simulink model "Drone2_simulink"  (R2024a)
settings: Solver=ode1be  StartTime=0.0  StopTime=1000  FixedStep=0.001  MaxStep=0.001  MinStep=0.00095  RelTol=1e-3
PreLoadFcn:
  | Drone_data;
model workspace: external: MATLAB File C:\Users\admin\OneDrive - Indian Institute of Technology Jodhpur\IIT JODHPUR\Research Work\Amphibious Drone\MATLAB_CODE\2025\New_Drone\Drone_1\Drone1_simulink_DataFile.m (data not in the file)
undefined symbols (not defined in the file): Environment, Newton, Raphson, Vehicle, X, Y, Z
libraries: sm_lib x1684, nesl_utility x63, slpidlib x25, eeGeneralControl x6, matrix_library x3, rllib x2, simulink x2, fl_lib x1, sharedutil x1, SignalEditorBlockLib x1
(part 4 of 17)

== system Drone2_simulink/Physical_system/Hydro Forces & Moments ==
  Bus Element In1 : Inport  PortName=HydroForces  Element=Drag.Forces
  Bus Element In2 : Inport  PortName=HydroForces  Element=Drag.Moments
  Bus Element In : Inport  PortName=HydroForces  Element=BuoyancyForce
  Bus Element In5 : Inport  PortName=HydroForces  Element=AddedMass.AMForcesXYZ
  Bus Element In6 : Inport  PortName=HydroForces  Element=AddedMass.AMMomentsXYZ
  Bus Element In7 : Inport  PortName=HydroForces  Element=AddedMass.CForcesXYZ
  Bus Element In8 : Inport  PortName=HydroForces  Element=AddedMass.CMomentsXYZ
  Bus Element In9 : Inport  PortName=HydroForces  Element=OceanCurrentForce
  Bus Element In11 : Inport  PortName=HydroForces  Element=WindForce
  Bus Element In10 : Inport  Port=2  PortName=CenterofMass  Element=Body.COM
  Added Mass Coriolis : Subsystem
  Added Mass Forces : Subsystem
  Buoyancy Force : Subsystem
  Lift and Drag Forces : Subsystem
  OceanCurrent Force : Subsystem
  Scope : Scope
  Scope1 : Scope
  Sum : Sum  Commented=on  Inputs=+++++
  Sum1 : Sum  Commented=on  Inputs=++++
  Wind force : Subsystem
  CoM : PMIOPort  Side=Left
  CoB : PMIOPort  Port=2  Side=Left
  wires:
  Bus Element In/1 -> Buoyancy Force/1(B)
  Bus Element In1/1 -> Sum/2, Lift and Drag Forces/1(Fxyz)
  Bus Element In2/1 -> Sum1/2, Lift and Drag Forces/3(Mxyz)
  Bus Element In5/1 -> Sum/3, Added Mass Forces/1(Fxyz)
  Bus Element In8/1 -> Sum1/4, Added Mass Coriolis/3(Mxyz)
  Bus Element In9/1 -> Sum/5, OceanCurrent Force/1(Ocean Current)
  Bus Element In10/1 -> Lift and Drag Forces/2(Centerofmass), Added Mass Coriolis/2(Centerofmass), Added Mass Forces/2(Centerofmass)
  Bus Element In6/1 -> Sum1/3, Added Mass Forces/3(Mxyz)
  Bus Element In7/1 -> Sum/4, Added Mass Coriolis/1(Fxyz)
  Bus Element In11/1 -> Wind force/1(Ocean Current)
  Sum/1 -> Scope/1
  Sum1/1 -> Scope1/1
  connections:
  CoB/RConn1 -- Buoyancy Force/RConn1
  Wind force/RConn1 -- OceanCurrent Force/RConn1 -- Added Mass Coriolis/RConn1 -- Added Mass Forces/RConn1 -- CoM/RConn1 -- Lift and Drag Forces/RConn1

== system Drone2_simulink/Physical_system/World ==
  Bottom floor : Subsystem  mask{ZB=-10, X=25, Z=0.1, Y=25, C1R=0.600, C1G=1, C1B=1.0, C2R=0, C2G=0.4, C2B=0.6}
      mask prompts: ZB "Distance of Bottom from World"; X "Length"; Z "Thikness"; Y "Width"; C1R "Red"; C1G "Green"; C1B "Blue"; C2R "Red"; C2G "Green"; C2B "Blue"
      mask init:
      | Color1 = [C1R C1G C1B];
      | Color2 = [C2R C2G C2B];
      mask DialogControl ParameterGroupVar Prompt: Bottom surface data
      mask DialogControl Container8 Prompt: Distance from World to Bottom
      mask DialogControl Container6 Prompt: Data of Each tiles
      mask DialogControl Container7 Prompt: Color 1
      mask DialogControl Container5 Prompt: Color2
      mask Display:
      | patch([0 10 10 0], [0 0 10 10], Color1);
      | patch([10 20 20 10], [0 0 10 10], Color2);
      | patch([0 10 10 0], [10 10 20 20], Color2);
      | patch([10 20 20 10], [10 10 20 20], Color1);
  MechanismConfiguration : sm_lib/Utilities/Mechanism Configuration  UniformGravity=Constant  GravityVector=[0 0 Environment.gravity]  GravityVectorUnits=m/s^2  LinearizationDelta=0.001  JointModeTransitionNonlinearIterations=2
  Solver Configuration : nesl_utility/Solver Configuration  PhysicalDomain=network_engine_domain  SubClassName=solver  LeftPortType=input  RightPortType=generic  Tones=[]  Harmonics=[]  SimulateNoise=off  Profile=off  UseLocalSampling=off  EnableSwitchedLinearOptims=on  FrequencyDomain=off  UseCCode=off  RelTol=0.001  AbsTol=0.001  MinStep=1e-09  ToWorkspace=off  RevertToSquareIcSolve=off  NumHomotopyIterations=100  PhasorMode=off  PhasorModeNumHarmonics=1  ConsistencySolver=NEWTON_XTOL_AFTER_FTOL  IndexReductionMethod=DerivativeReplacement  DoDC=off  ResidualTolerance=1e-09  ConsistencyTolSource=LOCAL  ConsistencyAbsTol=0.001  ConsistencyRelTol=0.001  ConsistencyTolFactor=0.001  UseLocalSolver=on  LocalSolverChoice=NE_BACKWARD_EULER_ADVANCER  ResolveIndetEquations=on  FunctionEvalNumThread=1  LocalSolverSampleTime=0.001  DoFixedCost=on  MaxNonlinIter=3  MaxModeIter=2  ComputeImpulses=off  ImpulseIterations=2  LinearAlgebra=Sparse  LinearAlgebraNumThread=0  EquationFormulation=NE_TIME_EF  DelaysMemoryBudget=1024  AutomaticFiltering=off  FilteringTimeConstant=0.001  PartitionStorageMethod=AS_NEEDED  PartitionMemoryBudget=1024  PartitionMethod=ROBUST  MultibodyUseLocalSolver=off  MultibodyLocalSolverChoice=ODE4  MultibodyLocalSolverSampleTime=0.001
  Spatial Contact Force : sm_lib/Forces and Torques/Spatial Contact Force  NormalForceType=SmoothSpringDamper  NormalStiffness=1  NormalStiffnessUnits=N/m  NormalDamping=0.001  NormalDampingUnits=N/(m/s)  NormalTransitionRegionWidth=0.05  NormalTransitionRegionWidthUnits=m  FrictionType=None  CoefficientOfStaticFriction=0  CoefficientOfDynamicFriction=0  FrictionalCriticalVelocity=1  FrictionalCriticalVelocityUnits=m/s  SenseContactSignal=off  SensePenetrationDepth=off  SenseSeparationDistance=off  SenseNormalForceMagnitude=off  SenseFrictionalForceMagnitude=off  SenseNormalVelocity=off  SenseTangentialVelocity=off  SenseContactBaseRotation=off  SenseContactBaseTranslation=off  SenseContactFollowerRotation=off  SenseContactFollowerTranslation=off  ZeroCrossDetectContactStartAndEnd=off
  Spatial Contact Force1 : sm_lib/Forces and Torques/Spatial Contact Force  NormalForceType=SmoothSpringDamper  NormalStiffness=1e2  NormalStiffnessUnits=N/m  NormalDamping=1e3  NormalDampingUnits=N/(m/s)  NormalTransitionRegionWidth=1e-4  NormalTransitionRegionWidthUnits=m  FrictionType=SmoothStickSlip  CoefficientOfStaticFriction=0.5  CoefficientOfDynamicFriction=0.3  FrictionalCriticalVelocity=1e-3  FrictionalCriticalVelocityUnits=m/s  SenseContactSignal=off  SensePenetrationDepth=off  SenseSeparationDistance=off  SenseNormalForceMagnitude=off  SenseFrictionalForceMagnitude=off  SenseNormalVelocity=off  SenseTangentialVelocity=off  SenseContactBaseRotation=off  SenseContactBaseTranslation=off  SenseContactFollowerRotation=off  SenseContactFollowerTranslation=off  ZeroCrossDetectContactStartAndEnd=off
  World : sm_lib/Frames and Transforms/World Frame
  water surface : sm_lib/Body Elements/Brick Solid  BrickDimensions=[500 500 0.01]  BrickDimensionsUnits=m  ExportEntireGeometry=on  InertiaType=CalculateFromGeometry  BasedOnType=Density  Density=1  DensityUnits=kg/m^3  Mass=1  MassUnits=kg  CenterOfMass=[0 0 0]  CenterOfMassUnits=m  MomentsOfInertia=[1 1 1]  MomentsOfInertiaUnits=kg*m^2  ProductsOfInertia=[0 0 0]  ProductsOfInertiaUnits=kg*m^2  GraphicType=FromGeometry  MarkerShape=Sphere  MarkerSize=10  GraphicVisPropType=SimpleVisualProperties  GraphicDiffuseColor=[0.0 0.8 1.0]  GraphicOpacity=0.1  GraphicSpecularColor=[0.5 0.5 0.5 1.0]  GraphicAmbientColor=[0.15 0.15 0.15 1.0]  GraphicEmissiveColor=[0.0 0.0 0.0 1.0]  GraphicShininess=75  DoExposeReferenceFrame=on  SerializedFrames=<Frames/>
  water surface ti bottom : sm_lib/Frames and Transforms/Rigid Transform  RotationMethod=None  FollAlignAxisA=+X  BaseAlignAxisA=+Y  FollAlignAxisB=+Y  BaseAlignAxisB=+Z  RotationStandardAxis=+Z  RotationAngle=0  RotationAngleUnits=deg  RotationArbitraryAxis=[0 0 1]  RotationSequenceAxes=FollowerAxes  RotationSequence=XYX  RotationSequenceAngles=[0 0 0]  RotationSequenceAnglesUnits=deg  RotationMatrix=[1 0 0;0 1 0;0 0 1]  Quaternion=[1 0 0 0]  TranslationMethod=Cartesian  TranslationCartesianOffset=[0 0 -8]  TranslationCartesianOffsetUnits=m  TranslationStandardAxis=+Z  TranslationStandardOffset=0  TranslationStandardOffsetUnits=m  TranslationROffset=0  TranslationROffsetUnits=m  TranslationThetaOffset=0  TranslationThetaOffsetUnits=deg  TranslationZOffset=0  TranslationZOffsetUnits=m
  surface : PMIOPort  Side=Right
  bottomsurf : PMIOPort  Port=2  Side=Right
  W : PMIOPort  Port=3  Side=Right
  connections:
  water surface/LConn1 -- Spatial Contact Force/LConn1
  surface/RConn1 -- Spatial Contact Force/RConn1
  bottomsurf/RConn1 -- Spatial Contact Force1/RConn1
  World/RConn1 -- water surface ti bottom/LConn1 -- Solver Configuration/RConn1 -- water surface/RConn1 -- MechanismConfiguration/RConn1 -- W/RConn1
  Bottom floor/LConn1 -- water surface ti bottom/RConn1
  Bottom floor/RConn1 -- Spatial Contact Force1/LConn1

== system Drone2_simulink/Visualization/psidot ==
  pqr : Inport
  phithetapsi : Inport  Port=2
  Mux1 : Mux  Inputs=[3 3 3]
  psidot : Fcn  Expr=(u[2]*u[4]+u[3]*u[7])/u[8]
  sincos : Trigonometry  Operator=sincos
  psid : Outport  Unit=rad/s  InitialOutput=0  VectorParamsAs1DForOutWhenUnconnected=off
  wires:
  sincos/2 -> Mux1/3
  sincos/1 -> Mux1/2
  phithetapsi/1 -> sincos/1
  pqr/1 -> Mux1/1
  Mux1/1 -> psidot/1
  psidot/1 -> psid/1

== system Drone2_simulink/Drive Controls/Thrust Controls/Depth and Pitch Control ==
  note: NOTE: Vehicle depth is indirectly controlled by the pitch angle which is regulated by the vertical thrusters ONLY
  PPf : Inport
  SPf : Inport  Port=2
  ZRef : Inport  Port=3
  Z : Inport  Port=4
  theta : Inport  Port=5
  Gain2 : Gain  Gain=-1
  Main Propellers Thrust Offset Compensation : Subsystem
  PDtheta : slpidlib/PID Controller  Controller=PD  Form=Parallel  TimeDomain=Continuous-time  UseExternalTs=off  SampleTime=-1  IntegratorMethod=Forward Euler  FilterMethod=Forward Euler  ControllerParametersSource=internal  P=-2023.58  I=1  UseKiTs=off  D=-2454.43  UseExternalDerivativeSource=off  N=3588.47  UseFilter=on  TunerSelectOption=Transfer Function Based (PID Tuner App)  InitialConditionSource=internal  InitialConditionForIntegrator=0  InitialConditionForFilter=0  DifferentiatorICPrevScaledInput=0  ExternalReset=none  TrackingMode=off  Kt=1  LimitOutput=off  SatLimitsSource=internal  UpperSaturationLimit=inf  LowerSaturationLimit=-inf  LinearizeAsGain=on  AntiWindupMode=none  Kb=1  LimitIntegrator=off  UpperIntegratorSaturationLimit=inf  LowerIntegratorSaturationLimit=-inf  POutMin=[]  POutMax=[]  IOutMin=[]  IOutMax=[]  DOutMin=[]  DOutMax=[]  NOutMin=[]  NOutMax=[]  SumOutMin=[]  SumOutMax=[]  SaturationOutMin=[]  SaturationOutMax=[]  PParamMin=[]  PParamMax=[]  IParamMin=[]  IParamMax=[]  DParamMin=[]  DParamMax=[]  NParamMin=[]  NParamMax=[]  KbParamMin=[]  KbParamMax=[]  KtParamMin=[]  KtParamMax=[]  KbOutMin=[]  KbOutMax=[]  KtOutMin=[]  KtOutMax=[]  IntegratorOutMin=[]  IntegratorOutMax=[]  FilterOutMin=[]  FilterOutMax=[]  SumI1OutMin=[]  SumI1OutMax=[]  SumI2OutMin=[]  SumI2OutMax=[]  SumI3OutMin=[]  SumI3OutMax=[]  SumI4OutMin=[]  SumI4OutMax=[]  SumDOutMin=[]  SumDOutMax=[]  DifferentiatorOutMin=[]  DifferentiatorOutMax=[]  FilterDiffOutCoefMin=[]  FilterDiffOutCoefMax=[]  ReciprocalOutMin=[]  ReciprocalOutMax=[]  SumDenOutMin=[]  SumDenOutMax=[]  SumNumOutMin=[]  SumNumOutMax=[]  DivideOutMin=[]  DivideOutMax=[]  UdiffTsProdOutMin=[]  UdiffTsProdOutMax=[]  NTsProdOutMin=[]  NTsProdOutMax=[]  UintegralTsProdOutMin=[]  UintegralTsProdOutMax=[]  UngainTsProdOutMin=[]  UngainTsProdOutMax=[]  ClampingZeroOutDataTypeStr=Inherit: Inherit via back propagation  ClampingZeroOutMin=[]  ClampingZeroOutMax=[]  FilterDenConstantOutDataTypeStr=Inherit: Inherit via back propagation  FilterDenConstantOutMin=[]  FilterDenConstantOutMax=[]  PCopyOutDataTypeStr=Inherit: Inherit via back propagation  PCopyOutMin=[]  PCopyOutMax=[]  NCopyOutDataTypeStr=Inherit: Inherit via back propagation  NCopyOutMin=[]  NCopyOutMax=[]  IntegratorContinuousStateAttributes=''  IntegratorStateMustResolveToSignalObject=off  IntegratorRTWStateStorageClass=Auto  FilterContinuousStateAttributes=''  FilterStateMustResolveToSignalObject=off  FilterRTWStateStorageClass=Auto  ParallelPVariant=InternalParameters  IdealPVariant=Disabled  IVariant=Disabled  DVariant=InternalParameters  IntegratorVariant=Disabled  SatVariant=Disabled  AWVariant=Disabled  PCopyVariant=Disabled  TRVariant=Disabled  FdbkBlocksVariant=Forward  IdealPFdbkVariant=Disabled  SatFdbkVariant=Disabled  DerivativeFilterVariant=ContFilter  NVariant=InternalParameters  NCopyVariant=Disabled  FilterICVariant=InternalICsFilter  IntegratorICVariant=Disabled  ExternalResetVariant=Disabled  TRSumVariant=Passthrough  SumFdbkVariant=Disabled  SumVariant=Sum_PD  TsampFilterVariant=InternalTs  TsampNgainVariant=Passthrough  TsampIntegralVariant=Disabled_SignalSpec  ExternalSaturationOutDataTypeStr=Inherit: Same as second input  DerivativeSourceVariant=ErrorSignal
  PIZ : slpidlib/PID Controller  Controller=PI  Form=Parallel  TimeDomain=Continuous-time  UseExternalTs=off  SampleTime=-1  IntegratorMethod=Forward Euler  FilterMethod=Forward Euler  ControllerParametersSource=internal  P=-0.25  I=-0.001  UseKiTs=off  D=0  UseExternalDerivativeSource=off  N=100  UseFilter=on  TunerSelectOption=Transfer Function Based (PID Tuner App)  InitialConditionSource=internal  InitialConditionForIntegrator=0  InitialConditionForFilter=0  DifferentiatorICPrevScaledInput=0  ExternalReset=none  TrackingMode=off  Kt=1  LimitOutput=off  SatLimitsSource=internal  UpperSaturationLimit=inf  LowerSaturationLimit=-inf  LinearizeAsGain=on  AntiWindupMode=none  Kb=1  LimitIntegrator=off  UpperIntegratorSaturationLimit=inf  LowerIntegratorSaturationLimit=-inf  POutMin=[]  POutMax=[]  IOutMin=[]  IOutMax=[]  DOutMin=[]  DOutMax=[]  NOutMin=[]  NOutMax=[]  SumOutMin=[]  SumOutMax=[]  SaturationOutMin=[]  SaturationOutMax=[]  PParamMin=[]  PParamMax=[]  IParamMin=[]  IParamMax=[]  DParamMin=[]  DParamMax=[]  NParamMin=[]  NParamMax=[]  KbParamMin=[]  KbParamMax=[]  KtParamMin=[]  KtParamMax=[]  KbOutMin=[]  KbOutMax=[]  KtOutMin=[]  KtOutMax=[]  IntegratorOutMin=[]  IntegratorOutMax=[]  FilterOutMin=[]  FilterOutMax=[]  SumI1OutMin=[]  SumI1OutMax=[]  SumI2OutMin=[]  SumI2OutMax=[]  SumI3OutMin=[]  SumI3OutMax=[]  SumI4OutMin=[]  SumI4OutMax=[]  SumDOutMin=[]  SumDOutMax=[]  DifferentiatorOutMin=[]  DifferentiatorOutMax=[]  FilterDiffOutCoefMin=[]  FilterDiffOutCoefMax=[]  ReciprocalOutMin=[]  ReciprocalOutMax=[]  SumDenOutMin=[]  SumDenOutMax=[]  SumNumOutMin=[]  SumNumOutMax=[]  DivideOutMin=[]  DivideOutMax=[]  UdiffTsProdOutMin=[]  UdiffTsProdOutMax=[]  NTsProdOutMin=[]  NTsProdOutMax=[]  UintegralTsProdOutMin=[]  UintegralTsProdOutMax=[]  UngainTsProdOutMin=[]  UngainTsProdOutMax=[]  ClampingZeroOutDataTypeStr=Inherit: Inherit via back propagation  ClampingZeroOutMin=[]  ClampingZeroOutMax=[]  FilterDenConstantOutDataTypeStr=Inherit: Inherit via back propagation  FilterDenConstantOutMin=[]  FilterDenConstantOutMax=[]  PCopyOutDataTypeStr=Inherit: Inherit via back propagation  PCopyOutMin=[]  PCopyOutMax=[]  NCopyOutDataTypeStr=Inherit: Inherit via back propagation  NCopyOutMin=[]  NCopyOutMax=[]  IntegratorContinuousStateAttributes=''  IntegratorStateMustResolveToSignalObject=off  IntegratorRTWStateStorageClass=Auto  FilterContinuousStateAttributes=''  FilterStateMustResolveToSignalObject=off  FilterRTWStateStorageClass=Auto  ParallelPVariant=InternalParameters  IdealPVariant=Disabled  IVariant=InternalParameters  DVariant=Disabled  IntegratorVariant=Continuous  SatVariant=Disabled  AWVariant=Passthrough  PCopyVariant=Disabled  TRVariant=Disabled  FdbkBlocksVariant=Forward  IdealPFdbkVariant=Disabled  SatFdbkVariant=Disabled  DerivativeFilterVariant=Disabled  NVariant=Disabled  NCopyVariant=Disabled_SignalSpec  FilterICVariant=Disabled  IntegratorICVariant=InternalICs  ExternalResetVariant=Disabled  TRSumVariant=Passthrough  SumFdbkVariant=Disabled  SumVariant=Sum_PI  TsampFilterVariant=InternalTs  TsampNgainVariant=Passthrough  TsampIntegralVariant=Disabled_SignalSpec  ExternalSaturationOutDataTypeStr=Inherit: Same as second input  DerivativeSourceVariant=Disabled
  Sum : Sum  Inputs=|+-
  Sum1 : Sum  Inputs=++|
  Sum2 : Sum  Inputs=|+-
  BVTfcmd : Outport
  SVTfcmd : Outport  Port=2
  wires:
  PPf/1 -> Main Propellers Thrust Offset Compensation/1(PPf)
  SPf/1 -> Main Propellers Thrust Offset Compensation/2(SPf)
  Gain2/1 -> SVTfcmd/1
  theta/1 -> Sum/2
  Sum/1 -> PDtheta/1
  PDtheta/1 -> Sum1/2
  Sum1/1 -> Gain2/1, BVTfcmd/1
  ZRef/1 -> Sum2/1
  Z/1 -> Sum2/2
  Sum2/1 -> PIZ/1
  PIZ/1 -> Sum/1
  Main Propellers Thrust Offset Compensation/1(VTf) -> Sum1/1

== system Drone2_simulink/Drive Controls/Thrust Controls/Heading and Yaw Control ==
  note: NOTE: Vehicle heading is regulated by the horizontal thrusters ONLY
  v : Inport
  psiRef : Inport  Port=2
  pqr : Inport  Port=3
  phithetapsi : Inport  Port=4
  Bus Selector : BusSelector  OutputSignals=psi
  Gain : Gain  Gain=-1
  PIDpsi : slpidlib/PID Controller  Controller=PID  Form=Parallel  TimeDomain=Continuous-time  UseExternalTs=off  SampleTime=-1  IntegratorMethod=Forward Euler  FilterMethod=Forward Euler  ControllerParametersSource=internal  P=564.0086345182  I=63718.733398644  UseKiTs=off  D=1.06148768314347  UseExternalDerivativeSource=off  N=71769.5968954127  UseFilter=on  TunerSelectOption=Transfer Function Based (PID Tuner App)  InitialConditionSource=internal  InitialConditionForIntegrator=0  InitialConditionForFilter=0  DifferentiatorICPrevScaledInput=0  ExternalReset=none  TrackingMode=off  Kt=1  LimitOutput=off  SatLimitsSource=internal  UpperSaturationLimit=inf  LowerSaturationLimit=-inf  LinearizeAsGain=on  AntiWindupMode=none  Kb=1  LimitIntegrator=off  UpperIntegratorSaturationLimit=inf  LowerIntegratorSaturationLimit=-inf  POutMin=[]  POutMax=[]  IOutMin=[]  IOutMax=[]  DOutMin=[]  DOutMax=[]  NOutMin=[]  NOutMax=[]  SumOutMin=[]  SumOutMax=[]  SaturationOutMin=[]  SaturationOutMax=[]  PParamMin=[]  PParamMax=[]  IParamMin=[]  IParamMax=[]  DParamMin=[]  DParamMax=[]  NParamMin=[]  NParamMax=[]  KbParamMin=[]  KbParamMax=[]  KtParamMin=[]  KtParamMax=[]  KbOutMin=[]  KbOutMax=[]  KtOutMin=[]  KtOutMax=[]  IntegratorOutMin=[]  IntegratorOutMax=[]  FilterOutMin=[]  FilterOutMax=[]  SumI1OutMin=[]  SumI1OutMax=[]  SumI2OutMin=[]  SumI2OutMax=[]  SumI3OutMin=[]  SumI3OutMax=[]  SumI4OutMin=[]  SumI4OutMax=[]  SumDOutMin=[]  SumDOutMax=[]  DifferentiatorOutMin=[]  DifferentiatorOutMax=[]  FilterDiffOutCoefMin=[]  FilterDiffOutCoefMax=[]  ReciprocalOutMin=[]  ReciprocalOutMax=[]  SumDenOutMin=[]  SumDenOutMax=[]  SumNumOutMin=[]  SumNumOutMax=[]  DivideOutMin=[]  DivideOutMax=[]  UdiffTsProdOutMin=[]  UdiffTsProdOutMax=[]  NTsProdOutMin=[]  NTsProdOutMax=[]  UintegralTsProdOutMin=[]  UintegralTsProdOutMax=[]  UngainTsProdOutMin=[]  UngainTsProdOutMax=[]  ClampingZeroOutDataTypeStr=Inherit: Inherit via back propagation  ClampingZeroOutMin=[]  ClampingZeroOutMax=[]  FilterDenConstantOutDataTypeStr=Inherit: Inherit via back propagation  FilterDenConstantOutMin=[]  FilterDenConstantOutMax=[]  PCopyOutDataTypeStr=Inherit: Inherit via back propagation  PCopyOutMin=[]  PCopyOutMax=[]  NCopyOutDataTypeStr=Inherit: Inherit via back propagation  NCopyOutMin=[]  NCopyOutMax=[]  IntegratorContinuousStateAttributes=''  IntegratorStateMustResolveToSignalObject=off  IntegratorRTWStateStorageClass=Auto  FilterContinuousStateAttributes=''  FilterStateMustResolveToSignalObject=off  FilterRTWStateStorageClass=Auto  ParallelPVariant=InternalParameters  IdealPVariant=Disabled  IVariant=InternalParameters  DVariant=InternalParameters  IntegratorVariant=Continuous  SatVariant=Disabled  AWVariant=Passthrough  PCopyVariant=Disabled  TRVariant=Disabled  FdbkBlocksVariant=Forward  IdealPFdbkVariant=Disabled  SatFdbkVariant=Disabled  DerivativeFilterVariant=ContFilter  NVariant=InternalParameters  NCopyVariant=Disabled  FilterICVariant=InternalICsFilter  IntegratorICVariant=InternalICs  ExternalResetVariant=Disabled  TRSumVariant=Passthrough  SumFdbkVariant=Disabled  SumVariant=Sum_PID  TsampFilterVariant=InternalTs  TsampNgainVariant=Passthrough  TsampIntegralVariant=Disabled_SignalSpec  ExternalSaturationOutDataTypeStr=Inherit: Same as second input  DerivativeSourceVariant=ErrorSignal
  PIDpsidot : slpidlib/PID Controller  Controller=PID  Form=Parallel  TimeDomain=Continuous-time  UseExternalTs=off  SampleTime=-1  IntegratorMethod=Forward Euler  FilterMethod=Forward Euler  ControllerParametersSource=internal  P=36876.176480623  I=4618545.3057506  UseKiTs=off  D=-22.9389890340326  UseExternalDerivativeSource=off  N=628  UseFilter=on  TunerSelectOption=Transfer Function Based (PID Tuner App)  InitialConditionSource=internal  InitialConditionForIntegrator=0  InitialConditionForFilter=0  DifferentiatorICPrevScaledInput=0  ExternalReset=none  TrackingMode=off  Kt=1  LimitOutput=off  SatLimitsSource=internal  UpperSaturationLimit=inf  LowerSaturationLimit=-inf  LinearizeAsGain=on  AntiWindupMode=none  Kb=1  LimitIntegrator=off  UpperIntegratorSaturationLimit=inf  LowerIntegratorSaturationLimit=-inf  POutMin=[]  POutMax=[]  IOutMin=[]  IOutMax=[]  DOutMin=[]  DOutMax=[]  NOutMin=[]  NOutMax=[]  SumOutMin=[]  SumOutMax=[]  SaturationOutMin=[]  SaturationOutMax=[]  PParamMin=[]  PParamMax=[]  IParamMin=[]  IParamMax=[]  DParamMin=[]  DParamMax=[]  NParamMin=[]  NParamMax=[]  KbParamMin=[]  KbParamMax=[]  KtParamMin=[]  KtParamMax=[]  KbOutMin=[]  KbOutMax=[]  KtOutMin=[]  KtOutMax=[]  IntegratorOutMin=[]  IntegratorOutMax=[]  FilterOutMin=[]  FilterOutMax=[]  SumI1OutMin=[]  SumI1OutMax=[]  SumI2OutMin=[]  SumI2OutMax=[]  SumI3OutMin=[]  SumI3OutMax=[]  SumI4OutMin=[]  SumI4OutMax=[]  SumDOutMin=[]  SumDOutMax=[]  DifferentiatorOutMin=[]  DifferentiatorOutMax=[]  FilterDiffOutCoefMin=[]  FilterDiffOutCoefMax=[]  ReciprocalOutMin=[]  ReciprocalOutMax=[]  SumDenOutMin=[]  SumDenOutMax=[]  SumNumOutMin=[]  SumNumOutMax=[]  DivideOutMin=[]  DivideOutMax=[]  UdiffTsProdOutMin=[]  UdiffTsProdOutMax=[]  NTsProdOutMin=[]  NTsProdOutMax=[]  UintegralTsProdOutMin=[]  UintegralTsProdOutMax=[]  UngainTsProdOutMin=[]  UngainTsProdOutMax=[]  ClampingZeroOutDataTypeStr=Inherit: Inherit via back propagation  ClampingZeroOutMin=[]  ClampingZeroOutMax=[]  FilterDenConstantOutDataTypeStr=Inherit: Inherit via back propagation  FilterDenConstantOutMin=[]  FilterDenConstantOutMax=[]  PCopyOutDataTypeStr=Inherit: Inherit via back propagation  PCopyOutMin=[]  PCopyOutMax=[]  NCopyOutDataTypeStr=Inherit: Inherit via back propagation  NCopyOutMin=[]  NCopyOutMax=[]  IntegratorContinuousStateAttributes=''  IntegratorStateMustResolveToSignalObject=off  IntegratorRTWStateStorageClass=Auto  FilterContinuousStateAttributes=''  FilterStateMustResolveToSignalObject=off  FilterRTWStateStorageClass=Auto  ParallelPVariant=InternalParameters  IdealPVariant=Disabled  IVariant=InternalParameters  DVariant=InternalParameters  IntegratorVariant=Continuous  SatVariant=Disabled  AWVariant=Passthrough  PCopyVariant=Disabled  TRVariant=Disabled  FdbkBlocksVariant=Forward  IdealPFdbkVariant=Disabled  SatFdbkVariant=Disabled  DerivativeFilterVariant=ContFilter  NVariant=InternalParameters  NCopyVariant=Disabled  FilterICVariant=InternalICsFilter  IntegratorICVariant=InternalICs  ExternalResetVariant=Disabled  TRSumVariant=Passthrough  SumFdbkVariant=Disabled  SumVariant=Sum_PID  TsampFilterVariant=InternalTs  TsampNgainVariant=Passthrough  TsampIntegralVariant=Disabled_SignalSpec  ExternalSaturationOutDataTypeStr=Inherit: Same as second input  DerivativeSourceVariant=ErrorSignal
  Sum : Sum  Inputs=-+|
  Sum1 : Sum  Inputs=-+|
  Sum2 : Sum  Inputs=++|
  Sum3 : Sum  Inputs=++|
  psidot : Subsystem
  side slip compensation : Subsystem
  BHTfcmd : Outport
  SHTfcmd : Outport  Port=2
  wires:
  pqr/1 -> psidot/1(pqr)
  phithetapsi/1 -> psidot/2(phithetapsi), Bus Selector/1
  psidot/1(psid) -> Sum/1
  Sum/1 -> PIDpsidot/1
  PIDpsidot/1 -> Gain/1, Sum2/2
  Sum1/1 -> PIDpsi/1
  PIDpsi/1 -> Sum/2
  Bus Selector/1 -> Sum1/1  "<psi>"
  psiRef/1 -> Sum1/2
  Sum2/1 -> BHTfcmd/1
  Gain/1 -> Sum3/2
  Sum3/1 -> SHTfcmd/1
  v/1 -> side slip compensation/1(v)
  side slip compensation/1(BHTf) -> Sum2/1
  side slip compensation/2(SHTf) -> Sum3/1

== system Drone2_simulink/Drive Controls/Thrust Controls/Longitudinal Speed (Surge) Control ==
  note: NOTE: Vehicle longitudinal speed is regulated by the main propellers ONLY
  uRef : Inport
  u : Inport  Port=2
  PIu : slpidlib/PID Controller  Controller=PI  Form=Parallel  TimeDomain=Continuous-time  UseExternalTs=off  SampleTime=-1  IntegratorMethod=Forward Euler  FilterMethod=Forward Euler  ControllerParametersSource=internal  P=78.8975  I=17.2606  UseKiTs=off  D=0  UseExternalDerivativeSource=off  N=100  UseFilter=on  TunerSelectOption=Transfer Function Based (PID Tuner App)  InitialConditionSource=internal  InitialConditionForIntegrator=0  InitialConditionForFilter=0  DifferentiatorICPrevScaledInput=0  ExternalReset=none  TrackingMode=off  Kt=1  LimitOutput=off  SatLimitsSource=internal  UpperSaturationLimit=inf  LowerSaturationLimit=-inf  LinearizeAsGain=on  AntiWindupMode=none  Kb=1  LimitIntegrator=off  UpperIntegratorSaturationLimit=inf  LowerIntegratorSaturationLimit=-inf  POutMin=[]  POutMax=[]  IOutMin=[]  IOutMax=[]  DOutMin=[]  DOutMax=[]  NOutMin=[]  NOutMax=[]  SumOutMin=[]  SumOutMax=[]  SaturationOutMin=[]  SaturationOutMax=[]  PParamMin=[]  PParamMax=[]  IParamMin=[]  IParamMax=[]  DParamMin=[]  DParamMax=[]  NParamMin=[]  NParamMax=[]  KbParamMin=[]  KbParamMax=[]  KtParamMin=[]  KtParamMax=[]  KbOutMin=[]  KbOutMax=[]  KtOutMin=[]  KtOutMax=[]  IntegratorOutMin=[]  IntegratorOutMax=[]  FilterOutMin=[]  FilterOutMax=[]  SumI1OutMin=[]  SumI1OutMax=[]  SumI2OutMin=[]  SumI2OutMax=[]  SumI3OutMin=[]  SumI3OutMax=[]  SumI4OutMin=[]  SumI4OutMax=[]  SumDOutMin=[]  SumDOutMax=[]  DifferentiatorOutMin=[]  DifferentiatorOutMax=[]  FilterDiffOutCoefMin=[]  FilterDiffOutCoefMax=[]  ReciprocalOutMin=[]  ReciprocalOutMax=[]  SumDenOutMin=[]  SumDenOutMax=[]  SumNumOutMin=[]  SumNumOutMax=[]  DivideOutMin=[]  DivideOutMax=[]  UdiffTsProdOutMin=[]  UdiffTsProdOutMax=[]  NTsProdOutMin=[]  NTsProdOutMax=[]  UintegralTsProdOutMin=[]  UintegralTsProdOutMax=[]  UngainTsProdOutMin=[]  UngainTsProdOutMax=[]  ClampingZeroOutDataTypeStr=Inherit: Inherit via back propagation  ClampingZeroOutMin=[]  ClampingZeroOutMax=[]  FilterDenConstantOutDataTypeStr=Inherit: Inherit via back propagation  FilterDenConstantOutMin=[]  FilterDenConstantOutMax=[]  PCopyOutDataTypeStr=Inherit: Inherit via back propagation  PCopyOutMin=[]  PCopyOutMax=[]  NCopyOutDataTypeStr=Inherit: Inherit via back propagation  NCopyOutMin=[]  NCopyOutMax=[]  IntegratorContinuousStateAttributes=''  IntegratorStateMustResolveToSignalObject=off  IntegratorRTWStateStorageClass=Auto  FilterContinuousStateAttributes=''  FilterStateMustResolveToSignalObject=off  FilterRTWStateStorageClass=Auto  ParallelPVariant=InternalParameters  IdealPVariant=Disabled  IVariant=InternalParameters  DVariant=Disabled  IntegratorVariant=Continuous  SatVariant=Disabled  AWVariant=Passthrough  PCopyVariant=Disabled  TRVariant=Disabled  FdbkBlocksVariant=Forward  IdealPFdbkVariant=Disabled  SatFdbkVariant=Disabled  DerivativeFilterVariant=Disabled  NVariant=Disabled  NCopyVariant=Disabled_SignalSpec  FilterICVariant=Disabled  IntegratorICVariant=InternalICs  ExternalResetVariant=Disabled  TRSumVariant=Passthrough  SumFdbkVariant=Disabled  SumVariant=Sum_PI  TsampFilterVariant=InternalTs  TsampNgainVariant=Passthrough  TsampIntegralVariant=Disabled_SignalSpec  ExternalSaturationOutDataTypeStr=Inherit: Same as second input  DerivativeSourceVariant=Disabled
  Sum : Sum  Inputs=|+-
  PPfcmd : Outport
  SPfcmd : Outport  Port=2
  wires:
  Sum/1 -> PIu/1
  PIu/1 -> PPfcmd/1, SPfcmd/1
  u/1 -> Sum/2
  uRef/1 -> Sum/1

== system Drone2_simulink/Hydrostatic & Hydrodynamic Effects/Added Mass Forces/Added Mass ==
  note: NOTE:
      | The forces due to added mass will me applied as external
      | forces, so they will oppose the direction of the accelerations
      |
      | $M_{rb}\dot{\nu}+C_{rb}(\nu)\nu= F_{propulsion} - M_a\dot{\nu}-C_a(\nu)\nu-D(\nu)\nu$
  Ma : Inport
  Abb : Inport  Port=2
  dwbdt : Inport  Port=3
  Demux : Demux  Outputs=[3,3]
  Gain : Gain  Gain=-1
  LPfilter : Subsystem
  Ma*[Abb,dwbdt]' : Product  Multiplication=Matrix(*)
  Reshape1 : Reshape  OutputDimensionality=Customize  OutputDimensions=[3,1]
  Reshape2 : Reshape  OutputDimensionality=Customize  OutputDimensions=[3,1]
  "[Abb,dwbdt]'" : Concatenate  Mode=Multidimensional array
  Fxyz : Outport
  Mxyz : Outport  Port=2
  wires:
  dwbdt/1 -> "[Abb,dwbdt]'"/2
  "[Abb,dwbdt]'"/1 -> Ma*[Abb,dwbdt]'/2
  Demux/2 -> Reshape2/1
  Ma/1 -> Ma*[Abb,dwbdt]'/1
  Abb/1 -> "[Abb,dwbdt]'"/1
  Demux/1 -> Reshape1/1
  Ma*[Abb,dwbdt]'/1 -> LPfilter/1(in)
  LPfilter/1(out) -> Gain/1
  Gain/1 -> Demux/1
  Reshape1/1 -> Fxyz/1
  Reshape2/1 -> Mxyz/1

== system Drone2_simulink/Hydrostatic & Hydrodynamic Effects/Added Mass Forces/Coriolis ==
  note: Coriolis matrix
  note: NOTE:
      | It is important to mention that the coriolis matrix due to added mass
      | computed here includes the de-stabilizing Munk-moment .
      | This moment acts to turn the vehicle perpendicular to the flow, and it
      | is most dominant for slender body vehicles in pitch and yaw when the
      | lateral velocities are non-zero.
      | This de-stabilizing effect will need to be accounted for in the design
      | of the control algorithm.
  Vb : Inport
  wb : Inport  Port=2
  Ma : Inport  Port=3
  Ca(V) : Subsystem
  Ca(V)*[Vb,wb]' : Product  Multiplication=Matrix(*)
  Demux : Demux  Outputs=6
  Demux1 : Demux  Outputs=[3,3]
  Gain : Gain  Gain=-1
  Ma*[Vb,wb]' : Product  Multiplication=Matrix(*)
  "[Vb,wb]'" : Concatenate  Mode=Multidimensional array
  Fxyz : Outport
  Mxyz : Outport  Port=2
  wires:
  Ma/1 -> Ma*[Vb,wb]'/1
  Vb/1 -> "[Vb,wb]'"/1
  wb/1 -> "[Vb,wb]'"/2
  "[Vb,wb]'"/1 -> Ca(V)*[Vb,wb]'/2, Ma*[Vb,wb]'/2
  Ma*[Vb,wb]'/1 -> Demux/1
  Demux/1 -> Ca(V)/1(a1)  "a1"
  Demux/2 -> Ca(V)/2(a2)  "a2"
  Demux/3 -> Ca(V)/3(a3)  "a3"
  Demux/4 -> Ca(V)/4(b1)  "b1"
  Demux/5 -> Ca(V)/5(b2)  "b2"
  Demux/6 -> Ca(V)/6(b3)  "b3"
  Ca(V)/1(Ca(V)) -> Ca(V)*[Vb,wb]'/1
  Ca(V)*[Vb,wb]'/1 -> Gain/1
  Demux1/1 -> Fxyz/1
  Demux1/2 -> Mxyz/1
  Gain/1 -> Demux1/1

== system Drone2_simulink/Hydrostatic & Hydrodynamic Effects/Drag Sub system/Aerodynamic drag ==
  Velocity : Inport
  Omega_b : Inport  Port=2
  Area : Subsystem
  Constant : Constant  Value=-Environment.Airdensity/2
  Linear drag : Constant  Value=diag([C_x C_y C_z])  mask{C_x=Vehicle.Air.Resistance.Cx, C_y=Vehicle.Air.Resistance.Cy, C_z=Vehicle.Air.Resistance.Cz}
      mask prompts: C_x "Drag X"; C_y "Drag Y"; C_z "Drag Z"
      mask DialogControl DescGroupVar Prompt: Drag
      mask DialogControl DescTextVar Prompt: Provide values for linear or rotation drage to formulate a diagonal  drag matrix
      mask Display: disp('diag([C_x C_y C_z])');
  MatrixMultiply{,1..3} (4 alike) : Product  Multiplication=Matrix(*)
  Reshape : Reshape  OutputDimensionality=Customize  OutputDimensions=[3,1]
  Reshape1 : Reshape  OutputDimensionality=Customize  OutputDimensions=[3,1]
  Rotational drag : Constant  Value=diag([C_x C_y C_z])  mask{C_x=Vehicle.Air.Resistance.Ck, C_y=Vehicle.Air.Resistance.Cm, C_z=Vehicle.Air.Resistance.Cn}
      mask prompts: C_x "Drag X"; C_y "Drag Y"; C_z "Drag Z"
      mask DialogControl DescGroupVar Prompt: Drag
      mask DialogControl DescTextVar Prompt: Provide values for linear or rotation drage to formulate a diagonal  drag matrix
      mask Display: disp('diag([C_x C_y C_z])');
  Subsystem : Subsystem
  Subsystem1 : Subsystem
  Force|_W : Outport
  Moment_W : Outport  Port=2
  wires:
  MatrixMultiply2/1 -> Force|_W/1
  Reshape1/1 -> MatrixMultiply3/2
  MatrixMultiply1/1 -> MatrixMultiply3/1
  Reshape/1 -> MatrixMultiply2/2
  MatrixMultiply/1 -> MatrixMultiply2/1
  Subsystem1/1(0.5rhov^2) -> Reshape1/1
  Area/2(Rotational) -> MatrixMultiply1/2
  Linear drag/1 -> MatrixMultiply/1
  Subsystem/1(0.5rhov^2) -> Reshape/1
  Rotational drag/1 -> MatrixMultiply1/1
  Area/1(Linear) -> MatrixMultiply/2
  Omega_b/1 -> Subsystem1/1(omega_b)
  Velocity/1 -> Subsystem/1(V_b)
  Constant/1 -> Subsystem1/2(rho), Subsystem/2(rho)
  MatrixMultiply3/1 -> Moment_W/1

== system Drone2_simulink/Hydrostatic & Hydrodynamic Effects/Drag Sub system/Hydrodyanamic drag ==
  Velocity : Inport
  Omega_b : Inport  Port=2
  Area : Subsystem
  Constant : Constant  Value=-Environment.Waterdensity/2
  Linear drag : Constant  Value=diag([C_x C_y C_z])  mask{C_x=Vehicle.Water.Resistance.Cx, C_y=Vehicle.Water.Resistance.Cy, C_z=Vehicle.Water.Resistance.Cz}
      mask prompts: C_x "Drag X"; C_y "Drag Y"; C_z "Drag Z"
      mask DialogControl DescGroupVar Prompt: Drag
      mask DialogControl DescTextVar Prompt: Provide values for linear or rotation drage to formulate a diagonal  drag matrix
      mask Display: disp('diag([C_x C_y C_z])');
  MATLAB Function : MATLAB Function  TreatAsAtomicUnit=on  mask{MIN=-5, MAX=5}
  MATLAB Function1 : MATLAB Function  TreatAsAtomicUnit=on  mask{A=-0.1, B=0.1}
      mask prompts: A "Min"; B "Max"
  MatrixMultiply{,1..3} (4 alike) : Product  Multiplication=Matrix(*)
  Reshape : Reshape  OutputDimensionality=Customize  OutputDimensions=[3,1]
  Reshape1 : Reshape  OutputDimensionality=Customize  OutputDimensions=[3,1]
  Rotational drag : Constant  Value=diag([C_x C_y C_z])  mask{C_x=Vehicle.Water.Resistance.Ck, C_y=Vehicle.Water.Resistance.Cm, C_z=Vehicle.Water.Resistance.Cn}
      mask prompts: C_x "Drag X"; C_y "Drag Y"; C_z "Drag Z"
      mask DialogControl DescGroupVar Prompt: Drag
      mask DialogControl DescTextVar Prompt: Provide values for linear or rotation drage to formulate a diagonal  drag matrix
      mask Display: disp('diag([C_x C_y C_z])');
  Scope : Scope
  Subsystem : Subsystem
  Subsystem1 : Subsystem
  Force|_W : Outport
  Moment_W : Outport  Port=2
  wires:
  Constant/1 -> Subsystem1/2(rho), Subsystem/2(rho)
  Velocity/1 -> Subsystem/1(V_b)
  Omega_b/1 -> Subsystem1/1(omega_b)
  Area/1(Linear) -> MatrixMultiply/2
  Rotational drag/1 -> MatrixMultiply1/1
  Linear drag/1 -> MatrixMultiply/1
  Area/2(Rotational) -> MatrixMultiply1/2
  Subsystem1/1(0.5rhov^2) -> Reshape1/1
  MatrixMultiply/1 -> MatrixMultiply2/1
  Reshape/1 -> MatrixMultiply2/2
  MatrixMultiply1/1 -> MatrixMultiply3/1
  Reshape1/1 -> MatrixMultiply3/2
  MatrixMultiply2/1 -> MATLAB Function/1(u)
  MatrixMultiply3/1 -> MATLAB Function1/1(u)
  Subsystem/1(0.5rhov^2) -> Scope/1, Reshape/1
  MATLAB Function/1(y) -> Force|_W/1
  MATLAB Function1/1(y) -> Moment_W/1

== system Drone2_simulink/Hydrostatic & Hydrodynamic Effects/Drag Sub system/Subsystem ==
  Altitude : Inport
  v : Inport  Port=2
  omega : Inport  Port=3
  Constant : Constant
  Subsystem : Subsystem
  Subsystem1 : Subsystem
  Subtract : Sum  Inputs=+-
  Transition Angular speed : Subsystem
  Transition data : Subsystem
  Transition speed : Subsystem
  1mwz : Outport
  W(z) : Outport  Port=2
  lambdav : Outport  Port=3
  lambdaomega : Outport  Port=4
  wires:
  Altitude/1 -> Transition data/1(Z)
  Subtract/1 -> 1mwz/1, Transition Angular speed/2(1mwz), Transition speed/2(1mwz)
  Constant/1 -> Subtract/1
  Transition data/1(W(z)) -> Subtract/2, W(z)/1, Transition Angular speed/1(W(z)), Transition speed/1(W(z))
  omega/1 -> Subsystem1/1(vector)
  Transition speed/1(lambdav) -> lambdav/1
  Transition Angular speed/1(lambdaomega) -> lambdaomega/1
  v/1 -> Subsystem/1(vector)
  Subsystem/1(Magnitude) -> Transition speed/3(vb)
  Subsystem1/1(Magnitude) -> Transition Angular speed/3(omegab)

== system Drone2_simulink/Hydrostatic & Hydrodynamic Effects/Ocean Current/Transition data ==
  Z : Inport
  Constant2 : Constant
  Exp : Math
  Gain : Gain  Gain=10/(Environment.Transition)
  Reciprocal : Product  Inputs=/
  Sum : Sum  Inputs=|++
  W(z) : Outport
  wires:
  Constant2/1 -> Sum/2
  Reciprocal/1 -> W(z)/1  "W(z)"
  Sum/1 -> Reciprocal/1
  Gain/1 -> Exp/1
  Z/1 -> Gain/1
  Exp/1 -> Sum/1

== system Drone2_simulink/Hydrostatic & Hydrodynamic Effects/Wind force/Transition data ==
  Z : Inport
  Constant2 : Constant
  Exp : Math
  Gain : Gain  Gain=10/(Environment.Transition)
  Reciprocal : Product  Inputs=/
  Sum : Sum  Inputs=|++
  W(z) : Outport
  wires:
  Constant2/1 -> Sum/2
  Reciprocal/1 -> W(z)/1  "W(z)"
  Sum/1 -> Reciprocal/1
  Gain/1 -> Exp/1
  Z/1 -> Gain/1
  Exp/1 -> Sum/1

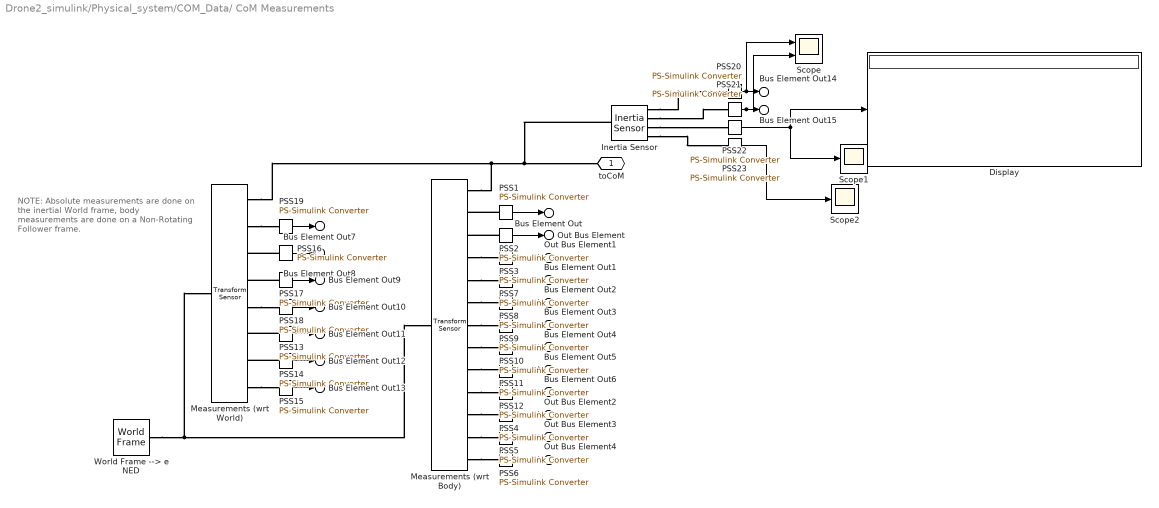
== system Drone2_simulink/Physical_system/COM_Data/ CoM Measurements ==
  note: NOTE:
      | Absolute measurements are done on the inertial World frame, body measurements are done on a Non-Rotating Follower frame.
  Display : Display
  Inertia Sensor : sm_lib/Body Elements/Inertia Sensor  SensorExtent=BodyGroup  SpanWeldJoints=off  ExcludeGroundedBodies=off  MeasurementFrame=Attached  SenseMass=on  SenseCenterOfMass=on  SenseInertiaMatrix=on  SenseCenteredInertiaMatrix=off  SensePrincipalInertiaMatrix=on  SenseRotationMatrix=off  GraphicType=PrincipalInertiaFrame  PrincipalInertiaFrameSize=20  GraphicVisPropType=SimpleVisualProperties  GraphicDiffuseColor=[1 0 1]  GraphicOpacity=1  GraphicSpecularColor=[0.5 0.5 0.5 1.0]  GraphicAmbientColor=[0.15 0.15 0.15 1.0]  GraphicEmissiveColor=[0.0 0.0 0.0 1.0]  GraphicShininess=75
  Measurements (wrt Body) : sm_lib/Frames and Transforms/Transform Sensor  MeasurementFrame=NonRotatingFollower  RotationSequence=XYX  SenseAngle=off  SenseAxis=off  SenseQ=off  SenseR=off  SenseRotationSequence=off  SenseOmegaX=on  SenseOmegaY=on  SenseOmegaZ=on  SenseOmega=off  SenseQDot=off  SenseRDot=off  SenseRotationSequenceDot=off  SenseAlphaX=on  SenseAlphaY=on  SenseAlphaZ=on  SenseAlpha=off  SenseQDDot=off  SenseRDDot=off  SenseX=off  SenseY=off  SenseZ=off  SenseXYZ=off  SenseRad=off  SenseAzim=off  SenseDist=off  SenseInc=off  SenseXDot=on  SenseYDot=on  SenseZDot=on  SenseXYZDot=off  SenseRadDot=off  SenseAzimDot=off  SenseDistDot=off  SenseIncDot=off  SenseXDDot=on  SenseYDDot=on  SenseZDDot=on  SenseXYZDDot=off  SenseRadDDot=off  SenseAzimDDot=off  SenseDistDDot=off  SenseIncDDot=off
  Measurements (wrt World) : sm_lib/Frames and Transforms/Transform Sensor  MeasurementFrame=World  RotationSequence=XYX  SenseAngle=off  SenseAxis=off  SenseQ=off  SenseR=on  SenseRotationSequence=off  SenseOmegaX=off  SenseOmegaY=off  SenseOmegaZ=off  SenseOmega=off  SenseQDot=off  SenseRDot=off  SenseRotationSequenceDot=off  SenseAlphaX=off  SenseAlphaY=off  SenseAlphaZ=off  SenseAlpha=off  SenseQDDot=off  SenseRDDot=off  SenseX=on  SenseY=on  SenseZ=on  SenseXYZ=off  SenseRad=off  SenseAzim=off  SenseDist=off  SenseInc=off  SenseXDot=on  SenseYDot=on  SenseZDot=on  SenseXYZDot=off  SenseRadDot=off  SenseAzimDot=off  SenseDistDot=off  SenseIncDot=off  SenseXDDot=off  SenseYDDot=off  SenseZDDot=off  SenseXYZDDot=off  SenseRadDDot=off  SenseAzimDDot=off  SenseDistDDot=off  SenseIncDDot=off
  PSS1 : nesl_utility/PS-Simulink Converter  PhysicalDomain=network_engine_domain  SubClassName=ps_output  LeftPortType=input  RightPortType=output  PseudoPeriodic=off  Frequencies=[]  VectorFormat=1-D array  Unit=rad/s  AffineConversion=off
  PSS{10..15} (6 alike) : nesl_utility/PS-Simulink Converter  PhysicalDomain=network_engine_domain  SubClassName=ps_output  LeftPortType=input  RightPortType=output  PseudoPeriodic=off  Frequencies=[]  VectorFormat=1-D array  Unit=m/s  AffineConversion=off
  PSS{16..18,21} (4 alike) : nesl_utility/PS-Simulink Converter  PhysicalDomain=network_engine_domain  SubClassName=ps_output  LeftPortType=input  RightPortType=output  PseudoPeriodic=off  Frequencies=[]  VectorFormat=1-D array  Unit=m  AffineConversion=off
  PSS19 : nesl_utility/PS-Simulink Converter  PhysicalDomain=network_engine_domain  SubClassName=ps_output  LeftPortType=input  RightPortType=output  PseudoPeriodic=off  Frequencies=[]  VectorFormat=1-D array  Unit=1  AffineConversion=off
  PSS2 : nesl_utility/PS-Simulink Converter  PhysicalDomain=network_engine_domain  SubClassName=ps_output  LeftPortType=input  RightPortType=output  PseudoPeriodic=off  Frequencies=[]  VectorFormat=1-D array  Unit=rad/s  AffineConversion=off
  PSS20 : nesl_utility/PS-Simulink Converter  PhysicalDomain=network_engine_domain  SubClassName=ps_output  LeftPortType=input  RightPortType=output  PseudoPeriodic=off  Frequencies=[]  VectorFormat=1-D array  Unit=kg  AffineConversion=off
  PSS22 : nesl_utility/PS-Simulink Converter  PhysicalDomain=network_engine_domain  SubClassName=ps_output  LeftPortType=input  RightPortType=output  PseudoPeriodic=off  Frequencies=[]  VectorFormat=1-D array  Unit=1  AffineConversion=on
  PSS23 : nesl_utility/PS-Simulink Converter  PhysicalDomain=network_engine_domain  SubClassName=ps_output  LeftPortType=input  RightPortType=output  PseudoPeriodic=off  Frequencies=[]  VectorFormat=1-D array  Unit=1  AffineConversion=on
  PSS3 : nesl_utility/PS-Simulink Converter  PhysicalDomain=network_engine_domain  SubClassName=ps_output  LeftPortType=input  RightPortType=output  PseudoPeriodic=off  Frequencies=[]  VectorFormat=1-D array  Unit=rad/s  AffineConversion=off
  PSS4 : nesl_utility/PS-Simulink Converter  PhysicalDomain=network_engine_domain  SubClassName=ps_output  LeftPortType=input  RightPortType=output  PseudoPeriodic=off  Frequencies=[]  VectorFormat=1-D array  Unit=m/s^2  AffineConversion=off
  PSS5 : nesl_utility/PS-Simulink Converter  PhysicalDomain=network_engine_domain  SubClassName=ps_output  LeftPortType=input  RightPortType=output  PseudoPeriodic=off  Frequencies=[]  VectorFormat=1-D array  Unit=m/s^2  AffineConversion=off
  PSS6 : nesl_utility/PS-Simulink Converter  PhysicalDomain=network_engine_domain  SubClassName=ps_output  LeftPortType=input  RightPortType=output  PseudoPeriodic=off  Frequencies=[]  VectorFormat=1-D array  Unit=m/s^2  AffineConversion=off
  PSS7 : nesl_utility/PS-Simulink Converter  PhysicalDomain=network_engine_domain  SubClassName=ps_output  LeftPortType=input  RightPortType=output  PseudoPeriodic=off  Frequencies=[]  VectorFormat=1-D array  Unit=rad/s^2  AffineConversion=off
  PSS8 : nesl_utility/PS-Simulink Converter  PhysicalDomain=network_engine_domain  SubClassName=ps_output  LeftPortType=input  RightPortType=output  PseudoPeriodic=off  Frequencies=[]  VectorFormat=1-D array  Unit=rad/s^2  AffineConversion=off
  PSS9 : nesl_utility/PS-Simulink Converter  PhysicalDomain=network_engine_domain  SubClassName=ps_output  LeftPortType=input  RightPortType=output  PseudoPeriodic=off  Frequencies=[]  VectorFormat=1-D array  Unit=rad/s^2  AffineConversion=off
  Scope : Scope  NumInputPorts=2
  Scope1 : Scope
  Scope2 : Scope
  World Frame --> e NED : sm_lib/Frames and Transforms/World Frame
  toCoM : PMIOPort  Side=Left
  Bus Element Out : Outport  PortName=Body  Element=wb.p
  Out Bus Element : Outport  PortName=Body  Element=wb.q
  Out Bus Element1 : Outport  PortName=Body  Element=wb.r
  Bus Element Out1 : Outport  PortName=Body  Element=dwbdt.pdot
  Bus Element Out2 : Outport  PortName=Body  Element=dwbdt.qdot
  Bus Element Out3 : Outport  PortName=Body  Element=dwbdt.rdot
  Bus Element Out4 : Outport  PortName=Body  Element=Vb.u
  Bus Element Out5 : Outport  PortName=Body  Element=Vb.v
  Bus Element Out6 : Outport  PortName=Body  Element=Vb.w
  Out Bus Element2 : Outport  PortName=Body  Element=Abe.ax
  Out Bus Element3 : Outport  PortName=Body  Element=Abe.ay
  Out Bus Element4 : Outport  PortName=Body  Element=Abe.az
  Bus Element Out14 : Outport  PortName=Body  Element=Mass
  Bus Element Out15 : Outport  PortName=Body  Element=COM
  Bus Element Out7 : Outport  Port=2  PortName=World  Element=R
  Bus Element Out8 : Outport  Port=2  PortName=World  Element=Xe.X
  Bus Element Out9 : Outport  Port=2  PortName=World  Element=Xe.Y
  Bus Element Out10 : Outport  Port=2  PortName=World  Element=Xe.Z
  Bus Element Out11 : Outport  Port=2  PortName=World  Element=Ve.Vx
  Bus Element Out12 : Outport  Port=2  PortName=World  Element=Ve.Vy
  Bus Element Out13 : Outport  Port=2  PortName=World  Element=Ve.Vz
  wires:
  PSS6/1 -> Out Bus Element4/1
  PSS5/1 -> Out Bus Element3/1
  PSS4/1 -> Out Bus Element2/1
  PSS3/1 -> Out Bus Element1/1
  PSS2/1 -> Out Bus Element/1
  PSS1/1 -> Bus Element Out/1
  PSS8/1 -> Bus Element Out2/1
  PSS9/1 -> Bus Element Out3/1
  PSS10/1 -> Bus Element Out4/1
  PSS11/1 -> Bus Element Out5/1
  PSS12/1 -> Bus Element Out6/1
  PSS13/1 -> Bus Element Out11/1
  PSS14/1 -> Bus Element Out12/1
  PSS15/1 -> Bus Element Out13/1
  PSS16/1 -> Bus Element Out8/1
  PSS18/1 -> Bus Element Out10/1
  PSS19/1 -> Bus Element Out7/1
  PSS17/1 -> Bus Element Out9/1
  PSS7/1 -> Bus Element Out1/1
  PSS20/1 -> Scope/1, Bus Element Out14/1
  PSS21/1 -> Scope/2, Bus Element Out15/1
  PSS22/1 -> Scope1/1, Display/1
  PSS23/1 -> Scope2/1
  connections:
  Measurements (wrt Body)/RConn4 -- PSS3/LConn1
  PSS2/LConn1 -- Measurements (wrt Body)/RConn3
  PSS1/LConn1 -- Measurements (wrt Body)/RConn2
  Measurements (wrt Body)/RConn1 -- Measurements (wrt World)/RConn1 -- Inertia Sensor/LConn1 -- toCoM/RConn1
  World Frame --> e NED/RConn1 -- Measurements (wrt World)/LConn1 -- Measurements (wrt Body)/LConn1
  Measurements (wrt Body)/RConn11 -- PSS4/LConn1
  Measurements (wrt Body)/RConn12 -- PSS5/LConn1
  Measurements (wrt Body)/RConn13 -- PSS6/LConn1
  Measurements (wrt Body)/RConn5 -- PSS7/LConn1
  Measurements (wrt Body)/RConn6 -- PSS8/LConn1
  Measurements (wrt Body)/RConn7 -- PSS9/LConn1
  Measurements (wrt Body)/RConn8 -- PSS10/LConn1
  Measurements (wrt Body)/RConn9 -- PSS11/LConn1
  Measurements (wrt Body)/RConn10 -- PSS12/LConn1
  PSS13/LConn1 -- Measurements (wrt World)/RConn6
  PSS14/LConn1 -- Measurements (wrt World)/RConn7
  Measurements (wrt World)/RConn8 -- PSS15/LConn1
  PSS16/LConn1 -- Measurements (wrt World)/RConn3
  PSS17/LConn1 -- Measurements (wrt World)/RConn4
  Measurements (wrt World)/RConn5 -- PSS18/LConn1
  Measurements (wrt World)/RConn2 -- PSS19/LConn1
  Inertia Sensor/RConn1 -- PSS20/LConn1
  Inertia Sensor/RConn2 -- PSS21/LConn1
  Inertia Sensor/RConn3 -- PSS22/LConn1
  Inertia Sensor/RConn4 -- PSS23/LConn1

== system Drone2_simulink/Physical_system/COM_Data/Derived Measurements ==
  Bus Element In1 : Inport  PortName=Body  Element=wb
  Bus Element In2 : Inport  PortName=Body  Element=Vb
  Bus Element In3 : Inport  PortName=Body  Element=Abe
  Bus Element In : Inport  Port=2  PortName=World  Element=R
  Body Acceleration : Subsystem
  Calculate DCM : Subsystem
  Euler Angles : Subsystem
  Incidence Angles : Subsystem
  Bus Element Out1 : Outport  PortName=Derived  Element=Euler.phi
  Bus Element Out2 : Outport  PortName=Derived  Element=Euler.theta
  Bus Element Out3 : Outport  PortName=Derived  Element=Euler.psi
  Bus Element Out4 : Outport  PortName=Derived  Element=Body.Abb
  Bus Element Out7 : Outport  PortName=Derived  Element=Body.V
  Bus Element Out5 : Outport  PortName=Derived  Element=Body.Incidences.alpha
  Bus Element Out6 : Outport  PortName=Derived  Element=Body.Incidences.beta
  Bus Element Out : Outport  PortName=Derived  Element=World.DCMbe
  wires:
  Bus Element In1/1 -> Euler Angles/1(pqr), Body Acceleration/1(wb)
  Euler Angles/1(phi) -> Bus Element Out1/1
  Euler Angles/2(theta) -> Bus Element Out2/1
  Euler Angles/3(psi) -> Bus Element Out3/1
  Bus Element In/1 -> Calculate DCM/1(R)
  Calculate DCM/1(DCMbe) -> Bus Element Out/1
  Bus Element In2/1 -> Incidence Angles/1(Vb), Body Acceleration/2(Vb)
  Bus Element In3/1 -> Body Acceleration/3(Abe)
  Incidence Angles/1(alpha) -> Bus Element Out5/1
  Incidence Angles/2(beta) -> Bus Element Out6/1
  Incidence Angles/3(V) -> Bus Element Out7/1
  Body Acceleration/1(Abb) -> Bus Element Out4/1
